simulink model "ConfiguredVirtualVehicleModel"  (R2023b)
settings: configuration reference "VehicleFixed05ms" (kept outside this file)
StartFcn:
  | %tic
StopFcn:
  | %toc
model workspace (MAT data in the model file):
  ExtDrvCmdsSwitch : Simulink.Parameter (value not decoded)
  ExtDrvRefSwitch : Simulink.Parameter (value not decoded)
  ExtEnvSwitch : Simulink.Parameter (value not decoded)
  ExtGndSwitch : Simulink.Parameter (value not decoded)
symbols that are objects in the model workspace (value not decoded): ExtDrvCmdsSwitch, ExtDrvRefSwitch, ExtEnvSwitch, ExtGndSwitch
undefined symbols (not defined in the file or in its folder): AccelCmd, AmbTemp, BaroPress, CtrlTcuInitGear, CtrlVcuCltch1InitCmd, CurvGradRef, CurvRef, DCM, DecelCmd, Disabled, DriverAeroRes, DriverDrivelineRes, DriverInitialGear, DriverPreviewDist, DriverRollRes, DriverShiftTime, DriverTimeConst, DriverTractiveForce, EnvAbsPrs, EnvAirTemp, EnvGrvty, EnvNomFrictionScaling, EnvNominalGrade, EnvWindVelX, EnvWindVelY, EnvWindVelZ, FTP75, Gnd, Grade, HazzardCmd, HighBeamCmd, lambda_mux, LeftSignalCmd, LngRef, LowBeamCmd, LtrRef, PhiRef, PlntVehDstCGFrntAxl, PlntVehDstCGRearAxl, PlntVehInitLatPos, PlntVehInitLongPos, PlntVehInitPitchAng, PlntVehInitRollAng, PlntVehInitVertPos, PlntVehInitYawAng, PlntVehMass, PlntVehTrckWdth, PlntVehYawMomentInertia, PlntWhlLdRadius, RightSignalCmd, ScnCRMaxLatAccel, ScnCRRadius, ScnDLCGateLongPos, ScnDLCLatRef, ScnDLCLatRefOffset, ScnDLCLongRefBpt, ScnDLCLongRefStartPos, ScnDLCVehicleWidth, ScnFHCounterDwellTime, ScnFHInitialDwellTime ... (+22)
libraries: simulink x27, autolibutils x8, vehdynlibscenariocommon x7, vehdynlibviscommon x3, vehdynlibdriver x2, sim3dgroundtruthsensorlib x2, autolibshared x2, vrlib x1, autolibsharedcommon x1, sharedtransform x1, sim3dlib x1, sim3dautolib x1
(part 6 of 6)

== system ConfiguredVirtualVehicleModel/Scenarios/Reference Generator/Reference Generator/Reference Generator/WOT ==
  "VehFdbk " : Inport
  Bus Creator : BusCreator  Inputs=3
  Bus Creator1 : BusCreator  Inputs=16
  Constant{,2..3,8,13..15,17} (8 alike) : Constant  Value=0
  Constant{1,4..7,9..12} (9 alike) : Constant  Value=false
  Constant16 : Constant  Value=zeros(1,3)
  Drive Cycle Source : autolibshared/Drive Cycle Source  cycleVar=Wide Open Throttle (WOT)  fileVar=L:\Bauto\matlab\test\toolbox\shared\autoblks\scenario\adac.txt  tfinal="2474  seconds"  cycleRepeat=off  outAccPort=off  outGearPort=off  gearList=No gear data  t_wot1=t_start  xdot_woto=0  xdot_wot1=xdot_r  t_wot2=t_wot2  xdot_wot2=0  t_wotend=simTime  srcUnit=mph  outUnit=mph  srcAccUnit=m/s/s  outAccUnit=m/s^2  dt=0  aMode=6  faultOption=off  velBnd=2  velBndUnit=mph  inUnit=m/s  timeBnd=1  failOption=off  stopSim=off  maxFaultCnt=10  maxFaultTime=2  maxTotFaultTime=15  traceOption=off  dtTrace=1  traceWindow=10  lastDCname=Custom Data Set  lastOutUnit=mph  lastDT=0  lastTB=1  lastSB=2  forceCalcBound=off
  Signal Specification : SignalSpecification  Unit=rad
  Signal Specification1 : SignalSpecification  Unit=one
  Signal Specification2 : SignalSpecification  Unit=one
  " Vis" : Outport  VectorParamsAs1DForOutWhenUnconnected=off
  " Ref" : Outport  Port=2  VectorParamsAs1DForOutWhenUnconnected=off
  " Fdbk" : Outport  Port=3  VectorParamsAs1DForOutWhenUnconnected=off
  wires:
  Constant2/1 -> Signal Specification2/1
  Constant8/1 -> Signal Specification1/1
  Constant4/1 -> Bus Creator1/7  "SteerHld"
  Signal Specification2/1 -> Bus Creator1/14  "DecelOvrCmd"
  Constant12/1 -> Bus Creator1/16  "DecelZero"
  Constant6/1 -> Bus Creator1/9  "EnblAccelOvr"
  Constant7/1 -> Bus Creator1/11  "AccelHld"
  Constant9/1 -> Bus Creator1/12  "AccelZero"
  Signal Specification1/1 -> Bus Creator1/10  "AccelOvrCmd"
  Constant11/1 -> Bus Creator1/15  "DecelHld"
  Constant10/1 -> Bus Creator1/13  "EnblDecelCmd"
  Constant5/1 -> Bus Creator1/8  "SteerZero"
  Signal Specification/1 -> Bus Creator1/6  "SteerOvrCmd"
  Constant3/1 -> Signal Specification/1
  Constant1/1 -> Bus Creator1/5  "EnblSteerCmd"
  Constant/1 -> Bus Creator1/2  "LtrlRef"
  Drive Cycle Source/1 -> Bus Creator1/1  "LngRef"
  Bus Creator1/1 -> " Ref"/1
  "VehFdbk "/1 -> " Fdbk"/1
  Bus Creator/1 -> " Vis"/1
  Constant15/1 -> Bus Creator/3  "ZRef"
  Constant14/1 -> Bus Creator/2  "YRef"
  Constant13/1 -> Bus Creator/1  "XRef"
  Constant16/1 -> Bus Creator1/3  "PoseRef"
  Constant17/1 -> Bus Creator1/4  "CurvRef"

== system ConfiguredVirtualVehicleModel/Environment/Ground Feedback/3D Engine/3D Engine Source/Multiple Points/For Each Subsystem ==
  phi,theta,psi : Inport  Partition=on  PartitionDimension=2  PartitionWidth=1  PartitionOffset=0
  For Each : ForEach  DisableCoverage=on
  Rotation Angles to Direction Cosine Matrix1 : sharedtransform/Rotation Angles to Direction Cosine Matrix  rotationOrder=YXZ  aMode=2
  Selector5 : Selector  InputPortWidth=3  IndexOptions=Index vector (dialog)  Indices=[2 1 3]  OutputSizes=1
  WheelDCM : Outport  ConcatenationDimension=3
  wires:
  Selector5/1 -> Rotation Angles to Direction Cosine Matrix1/1
  Rotation Angles to Direction Cosine Matrix1/1 -> WheelDCM/1
  phi,theta,psi/1 -> Selector5/1

== system ConfiguredVirtualVehicleModel/Scenarios/Reference Generator/Reference Generator/3D Engine/3D Engine/Part Rotation Concatenation ==
  Body Roll : Inport
  Body Ptich : Inport  Port=2
  Body Yaw : Inport  Port=3
  WheelFrontLeft Pitch : Inport  Port=4
  WheelFrontRight Pitch : Inport  Port=5
  WheelRearLeft Pitch : Inport  Port=6
  WheelRearRight Ptich : Inport  Port=7
  WheelFrontLeft Roll : Inport  Port=8
  WheelFrontRight Roll : Inport  Port=9
  WheelRearLeft Roll : Inport  Port=10
  WheelRearRight Roll : Inport  Port=11
  WheelFrontLeft Yaw : Inport  Port=12
  WheelFrontRight Yaw : Inport  Port=13
  WheelRearLeft Yaw : Inport  Port=14
  WheelRearRight Yaw : Inport  Port=15
  AllParts : Concatenate  NumInputs=5  Mode=Multidimensional array
  Body : Concatenate  NumInputs=3  Mode=Multidimensional array  ConcatenateDimension=2
  WheelFrontLeft : Concatenate  NumInputs=3  Mode=Multidimensional array  ConcatenateDimension=2
  WheelFrontRight : Concatenate  NumInputs=3  Mode=Multidimensional array  ConcatenateDimension=2
  WheelRearLeft : Concatenate  NumInputs=3  Mode=Multidimensional array  ConcatenateDimension=2
  WheelRearRight : Concatenate  NumInputs=3  Mode=Multidimensional array  ConcatenateDimension=2
  ConcatOut : Outport  VectorParamsAs1DForOutWhenUnconnected=off
  wires:
  WheelRearRight Roll/1 -> WheelRearRight/1
  WheelRearRight Ptich/1 -> WheelRearRight/2
  WheelRearLeft Roll/1 -> WheelRearLeft/1
  WheelRearLeft Pitch/1 -> WheelRearLeft/2
  WheelFrontRight Roll/1 -> WheelFrontRight/1
  WheelFrontRight Pitch/1 -> WheelFrontRight/2
  WheelFrontLeft Roll/1 -> WheelFrontLeft/1
  WheelFrontLeft Pitch/1 -> WheelFrontLeft/2
  Body Roll/1 -> Body/1
  Body Ptich/1 -> Body/2
  WheelFrontRight Yaw/1 -> WheelFrontRight/3
  WheelRearRight/1 -> AllParts/5
  AllParts/1 -> ConcatOut/1
  WheelRearLeft Yaw/1 -> WheelRearLeft/3
  WheelRearRight Yaw/1 -> WheelRearRight/3
  WheelFrontRight/1 -> AllParts/3
  WheelRearLeft/1 -> AllParts/4
  Body/1 -> AllParts/1
  WheelFrontLeft/1 -> AllParts/2
  WheelFrontLeft Yaw/1 -> WheelFrontLeft/3
  Body Yaw/1 -> Body/3

== system ConfiguredVirtualVehicleModel/Scenarios/Reference Generator/Reference Generator/3D Engine/3D Engine/Part Translation Concatenation ==
  BodyX : Inport
  BodyY : Inport  Port=2
  BodyZ : Inport  Port=3
  WheelFrontLeftX : Inport  Port=4
  WheelFrontRightX : Inport  Port=5
  WheelRearLeftX : Inport  Port=6
  WheelRearRightX : Inport  Port=7
  WheelFrontLeftY : Inport  Port=8
  WheelFrontRightY : Inport  Port=9
  WheelRearLeftY : Inport  Port=10
  WheelRearRightY : Inport  Port=11
  WheelFrontLeftZ : Inport  Port=12
  WheelFrontRightZ : Inport  Port=13
  WheelRearLeftZ : Inport  Port=14
  WheelRearRightZ : Inport  Port=15
  AllParts : Concatenate  NumInputs=5  Mode=Multidimensional array
  Body : Concatenate  NumInputs=3  Mode=Multidimensional array  ConcatenateDimension=2
  WheelFrontLeft : Concatenate  NumInputs=3  Mode=Multidimensional array  ConcatenateDimension=2
  WheelFrontRight : Concatenate  NumInputs=3  Mode=Multidimensional array  ConcatenateDimension=2
  WheelRearLeft : Concatenate  NumInputs=3  Mode=Multidimensional array  ConcatenateDimension=2
  WheelRearRight : Concatenate  NumInputs=3  Mode=Multidimensional array  ConcatenateDimension=2
  ConcatOut : Outport  VectorParamsAs1DForOutWhenUnconnected=off
  wires:
  WheelFrontRightZ/1 -> WheelFrontRight/3
  WheelRearLeftX/1 -> WheelRearLeft/1
  WheelRearRight/1 -> AllParts/5
  WheelRearLeftY/1 -> WheelRearLeft/2
  AllParts/1 -> ConcatOut/1
  WheelRearLeftZ/1 -> WheelRearLeft/3
  WheelRearRightY/1 -> WheelRearRight/2
  WheelFrontRightX/1 -> WheelFrontRight/1
  WheelFrontRightY/1 -> WheelFrontRight/2
  WheelRearRightZ/1 -> WheelRearRight/3
  WheelFrontRight/1 -> AllParts/3
  WheelRearLeft/1 -> AllParts/4
  Body/1 -> AllParts/1
  WheelRearRightX/1 -> WheelRearRight/1
  WheelFrontLeft/1 -> AllParts/2
  BodyY/1 -> Body/2
  WheelFrontLeftY/1 -> WheelFrontLeft/2
  WheelFrontLeftZ/1 -> WheelFrontLeft/3
  WheelFrontLeftX/1 -> WheelFrontLeft/1
  BodyZ/1 -> Body/3
  BodyX/1 -> Body/1

== system ConfiguredVirtualVehicleModel/Scenarios/Reference Generator/Reference Generator/3D Engine/3D Engine/Scale ==
  Constant{1..12,17,32..33} (15 alike) : Constant  OutDataTypeStr=single
  PartConcatenation : Subsystem
  ScaleOut : Outport  VectorParamsAs1DForOutWhenUnconnected=off
  wires:
  PartConcatenation/1(ConcatOut) -> ScaleOut/1
  Constant12/1 -> PartConcatenation/1(BodyX)
  Constant17/1 -> PartConcatenation/2(BodyY)
  Constant32/1 -> PartConcatenation/3(BodyZ)
  Constant33/1 -> PartConcatenation/4(WheelFrontLeftX)
  Constant1/1 -> PartConcatenation/5(WheelFrontLeftY)
  Constant2/1 -> PartConcatenation/6(WheelFrontLeftZ)
  Constant5/1 -> PartConcatenation/7(WheelFrontRightX)
  Constant3/1 -> PartConcatenation/8(WheelFrontRightY)
  Constant4/1 -> PartConcatenation/9(WheelFrontRightZ)
  Constant8/1 -> PartConcatenation/10(WheelRearLeftX)
  Constant6/1 -> PartConcatenation/11(WheelRearLeftY)
  Constant7/1 -> PartConcatenation/12(WheelRearLeftZ)
  Constant11/1 -> PartConcatenation/13(WheelRearRightX)
  Constant9/1 -> PartConcatenation/14(WheelRearRightY)
  Constant10/1 -> PartConcatenation/15(WheelRearRightZ)

== system ConfiguredVirtualVehicleModel/Scenarios/Reference Generator/Reference Generator/3D Engine/3D Engine/Scale/PartConcatenation ==
  BodyX : Inport
  BodyY : Inport  Port=2
  BodyZ : Inport  Port=3
  WheelFrontLeftX : Inport  Port=4
  WheelFrontLeftY : Inport  Port=5
  WheelFrontLeftZ : Inport  Port=6
  WheelFrontRightX : Inport  Port=7
  WheelFrontRightY : Inport  Port=8
  WheelFrontRightZ : Inport  Port=9
  WheelRearLeftX : Inport  Port=10
  WheelRearLeftY : Inport  Port=11
  WheelRearLeftZ : Inport  Port=12
  WheelRearRightX : Inport  Port=13
  WheelRearRightY : Inport  Port=14
  WheelRearRightZ : Inport  Port=15
  AllParts : Concatenate  NumInputs=5  Mode=Multidimensional array
  Body : Concatenate  NumInputs=3  Mode=Multidimensional array  ConcatenateDimension=2
  WheelFrontLeft : Concatenate  NumInputs=3  Mode=Multidimensional array  ConcatenateDimension=2
  WheelFrontRight : Concatenate  NumInputs=3  Mode=Multidimensional array  ConcatenateDimension=2
  WheelRearLeft : Concatenate  NumInputs=3  Mode=Multidimensional array  ConcatenateDimension=2
  WheelRearRight : Concatenate  NumInputs=3  Mode=Multidimensional array  ConcatenateDimension=2
  ConcatOut : Outport  VectorParamsAs1DForOutWhenUnconnected=off
  wires:
  WheelFrontRightZ/1 -> WheelFrontRight/3
  WheelRearLeftX/1 -> WheelRearLeft/1
  WheelRearRight/1 -> AllParts/5
  WheelRearLeftY/1 -> WheelRearLeft/2
  AllParts/1 -> ConcatOut/1
  WheelRearLeftZ/1 -> WheelRearLeft/3
  WheelRearRightY/1 -> WheelRearRight/2
  WheelFrontRightX/1 -> WheelFrontRight/1
  WheelFrontRightY/1 -> WheelFrontRight/2
  WheelRearRightZ/1 -> WheelRearRight/3
  WheelFrontRight/1 -> AllParts/3
  WheelRearLeft/1 -> AllParts/4
  Body/1 -> AllParts/1
  WheelRearRightX/1 -> WheelRearRight/1
  WheelFrontLeft/1 -> AllParts/2
  BodyY/1 -> Body/2
  WheelFrontLeftY/1 -> WheelFrontLeft/2
  WheelFrontLeftZ/1 -> WheelFrontLeft/3
  WheelFrontLeftX/1 -> WheelFrontLeft/1
  BodyZ/1 -> Body/3
  BodyX/1 -> Body/1
